simulink model "Velocity_estimator_Mclab_new"  (R2017a)
settings: Solver=VariableStepAuto  StartTime=0.0  StopTime=10.0  RelTol=1e-3
settings Model: Creator=torees  LastModifiedBy=torees

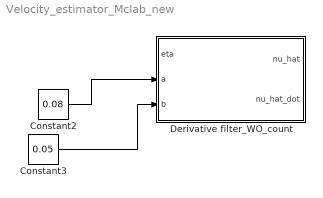
== system Velocity_estimator_Mclab_new ==
  Constant2 : Constant  Value=0.08
  Constant3 : Constant  Value=0.05
  Derivative filter_WO_count : Subsystem
  wires:
  Constant3/1 -> Derivative filter_WO_count/3(b)
  Constant2/1 -> Derivative filter_WO_count/2(a)

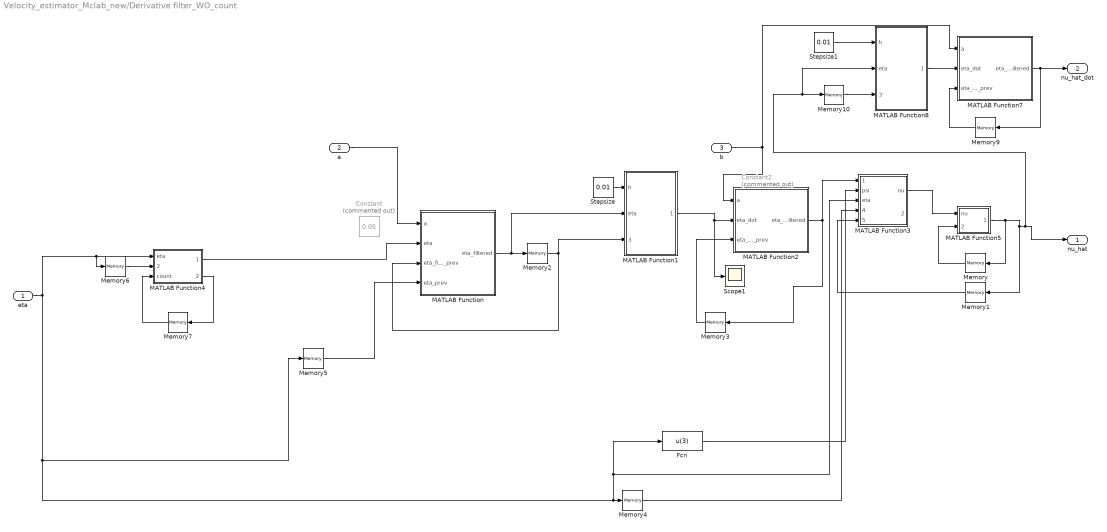
== system Velocity_estimator_Mclab_new/Derivative filter_WO_count ==
  eta : Inport
  a : Inport  Port=2
  b : Inport  Port=3
  Constant : Constant  Commented=on  Value=0.05
  Constant2 : Constant  Commented=on  Value=0.03
  Fcn : Fcn  Expr=u(3)
  MATLAB Function : MATLAB Function  TreatAsAtomicUnit=on
  MATLAB Function1 : MATLAB Function  TreatAsAtomicUnit=on
  MATLAB Function2 : MATLAB Function  TreatAsAtomicUnit=on
  MATLAB Function3 : MATLAB Function  TreatAsAtomicUnit=on
  MATLAB Function4 : MATLAB Function  TreatAsAtomicUnit=on
  MATLAB Function5 : MATLAB Function  TreatAsAtomicUnit=on
  MATLAB Function7 : MATLAB Function  TreatAsAtomicUnit=on
  MATLAB Function8 : MATLAB Function  TreatAsAtomicUnit=on
  Memory{,1..6,9..10} (9 alike) : Memory  X0=[0 0 0]
  Memory7 : Memory
  Scope1 : Scope
  Stepsize : Constant  Value=0.01
  Stepsize1 : Constant  Value=0.01
  nu_hat : Outport
  nu_hat_dot : Outport  Port=2
  wires:
  MATLAB Function7/1(eta_dot_filtered) -> Memory9/1, nu_hat_dot/1
  MATLAB Function4/2(count_out) -> Memory7/1
  Memory7/1 -> MATLAB Function4/3(count)
  Memory6/1 -> MATLAB Function4/2(eta_prev)
  MATLAB Function4/1(eta_out) -> MATLAB Function/2(eta)
  Stepsize1/1 -> MATLAB Function8/1(h)
  Memory10/1 -> MATLAB Function8/3(eta_prev)
  MATLAB Function8/1(eta_dot) -> MATLAB Function7/2(eta_dot)
  Memory9/1 -> MATLAB Function7/3(eta_dot_filtered_prev)
  eta/1 -> MATLAB Function4/1(eta), Memory6/1, Memory4/1, MATLAB Function3/3(eta), Fcn/1, Memory5/1
  Memory5/1 -> MATLAB Function/4(eta_prev)
  MATLAB Function3/1(nu) -> MATLAB Function5/1(nu)
  Memory4/1 -> MATLAB Function3/4(prev_eta)
  Memory1/1 -> MATLAB Function3/5(prev_nu)
  MATLAB Function/1(eta_filtered) -> Memory2/1, MATLAB Function1/2(eta)
  b/1 -> MATLAB Function2/1(a), MATLAB Function7/1(a)
  a/1 -> MATLAB Function/1(a)
  Memory3/1 -> MATLAB Function2/3(eta_dot_filtered_prev)
  MATLAB Function2/1(eta_dot_filtered) -> MATLAB Function3/1(eta_dot), Memory3/1
  MATLAB Function1/1(eta_dot) -> MATLAB Function2/2(eta_dot), Scope1/1
  Memory2/1 -> MATLAB Function/3(eta_filtered_prev), MATLAB Function1/3(eta_prev)
  Stepsize/1 -> MATLAB Function1/1(h)
  Fcn/1 -> MATLAB Function3/2(psi)
  MATLAB Function5/1(nu_out) -> Memory/1, Memory1/1, nu_hat/1, Memory10/1, MATLAB Function8/2(eta)
  Memory/1 -> MATLAB Function5/2(nu_prev)

== matlab function Velocity_estimator_Mclab_new/Derivative filter_WO_count/MATLAB Function5 ==
  data: nu input; nu_out output; nu_prev input
function nu_out = fcn(nu, nu_prev)
nu_out = nu;
% max aks 0.13 m/s^2 eller 0.0136 per timestep(10hz)
% max aks 0.0267 m/s^2 eller 0.00267 per timestep(10hz)
tilde_nu_x =abs(nu(1)) - abs(nu_prev(1));
tilde_nu_y =abs(nu(2)) - abs(nu_prev(2));
tilde_nu_yaw =abs(nu(3)) - abs(nu_prev(3));

a_x =0.00136*0.8;
a_y =0.000267*1.7;
a_yaw =deg2rad(0.061/1.5);


if (tilde_nu_x > a_x) 
    if sign(nu(1)) == 1
        nu_out(1) = nu_prev(1) + a_x;
    end
    if sign(nu(1)) == -1
        nu_out(1) = nu_prev(1) - a_x;
    end
    
end
if (tilde_nu_y > a_y) 
    if sign(nu(2)) == 1
        nu_out(2) = nu_prev(2) + a_y;
    end
    if sign(nu(2)) == -1
        nu_out(2) = nu_prev(2) - a_y;
    end
    
end

if (tilde_nu_yaw > a_yaw) 
    if sign(nu(3)) == 1
        nu_out(3) = nu_prev(3) + a_yaw;
    end
    if sign(nu(3)) == -1
        nu_out(3) = nu_prev(3) - a_yaw;
    end
    
end

== matlab function Velocity_estimator_Mclab_new/Derivative filter_WO_count/MATLAB Function ==
  data: a input; eta_filtered output; eta input; eta_filtered_prev input; eta_prev input
function eta_filtered  = fcn(a,eta,eta_filtered_prev,eta_prev)

psi = eta(3);
psitilde = psi-eta_prev(3);


eta_filtered = a*eta + (1-a)*eta_filtered_prev;

== matlab function Velocity_estimator_Mclab_new/Derivative filter_WO_count/MATLAB Function1 ==
  data: h input; eta_dot output; eta input; eta_prev input
function eta_dot  = fcn(h,eta,eta_prev)

eta_tilde = eta-eta_prev;
eta_dot = (eta_tilde)./h;

if eta_dot(3)>6;
    eta_dot(3)=5;
elseif eta_dot(3)<-6;
   eta_dot(3)=-6; 
end

== matlab function Velocity_estimator_Mclab_new/Derivative filter_WO_count/MATLAB Function2 ==
  data: a input; eta_dot_filtered output; eta_dot input; eta_dot_filtered_prev input
function eta_dot_filtered = fcn(a,eta_dot,eta_dot_filtered_prev)

eta_dot_filtered = a*eta_dot + (1-a)*eta_dot_filtered_prev;

== matlab function Velocity_estimator_Mclab_new/Derivative filter_WO_count/MATLAB Function3 ==
  data: eta_dot input; nu output; psi input; eta input; prev_eta input; prev_nu input; count_out output
function [nu,count_out] = fcn(eta_dot,psi,eta,prev_eta,prev_nu)
%eta_dot(1) max 0.4 m/s
%eta_dot(2) max 0.11 m/s
%eta_dot(3) max 6.1 rad/s




if(prev_eta(1)==eta(1)||prev_eta(2)==eta(2)||prev_eta(3)==eta(3))
    nu = prev_nu;
    count_out =1;
else
    %if count == 1
        %nu = prev_nu;
        %count_out = 0;
    %else
        R_inv = [cos(psi)  sin(psi) 0
                 -sin(psi) cos(psi) 0
                 0         0        1];
        nu = R_inv*eta_dot;
        count_out = 0;
    %end
end

== matlab function Velocity_estimator_Mclab_new/Derivative filter_WO_count/MATLAB Function4 ==
  data: eta input; eta_out output; eta_prev input; count input; count_out output
function [eta_out,count_out] = fcn(eta,eta_prev,count)

angle_d = eta(3)*180/pi;%+count*360;
angle = eta_prev(3)*180/pi;%+count*360;

angle_tilde = angle_d-angle;

if abs(angle_tilde)>300;
    count_out=-sign(angle_tilde)+count;
    angle_out=angle_d+count_out*360;
else
    count_out=count;
    angle_out=angle_d+count_out*360;
end

eta_out = eta;
eta_out(3) = angle_out*pi/180;


end

== matlab function Velocity_estimator_Mclab_new/Derivative filter_WO_count/MATLAB Function7 ==
  data: a input; eta_dot_filtered output; eta_dot input; eta_dot_filtered_prev input
function eta_dot_filtered = fcn(a,eta_dot,eta_dot_filtered_prev)

eta_dot_filtered = a*eta_dot + (1-a)*eta_dot_filtered_prev;

== matlab function Velocity_estimator_Mclab_new/Derivative filter_WO_count/MATLAB Function8 ==
  data: h input; eta_dot output; eta input; eta_prev input
function eta_dot  = fcn(h,eta,eta_prev)

eta_tilde = eta-eta_prev;
eta_dot = (eta_tilde)./h;

if eta_dot(3)>5;
    eta_dot(3)=5;
elseif eta_dot(3)<-5;
   eta_dot(3)=-5; 
end
